simulink model "lunar_lander_sim_PWPF_transferMatrix_2023a"  (R2023a)
settings: Solver=FixedStepAuto  StartTime=0  StopTime=200  FixedStep=0.001  RelTol=1e-3
values from neighbouring files (symbols this model uses):
  D = Y_bar(:,1:m)    [Auxi_OKID_JXL.m]    (also in limit_cycle_est.m = 0:0.01:1)
undefined symbols (not defined in the file or in its folder): aMode
libraries: simulink_extras x8, slpidlib x6, shared6dofsys x2, sharedutil x2
settings Model: Creator=cnsl  LastModifiedBy=s3928

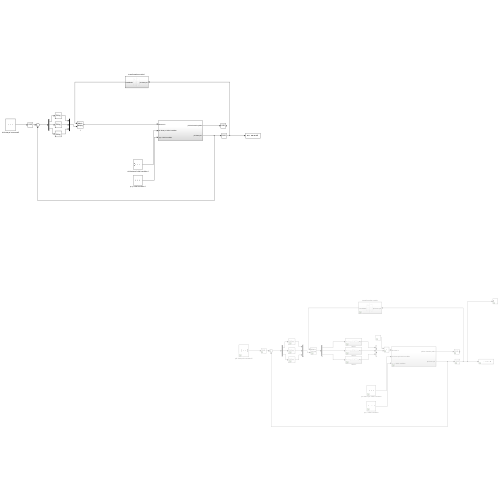
[thumbnail: Simulink's stored preview of the top-level diagram]
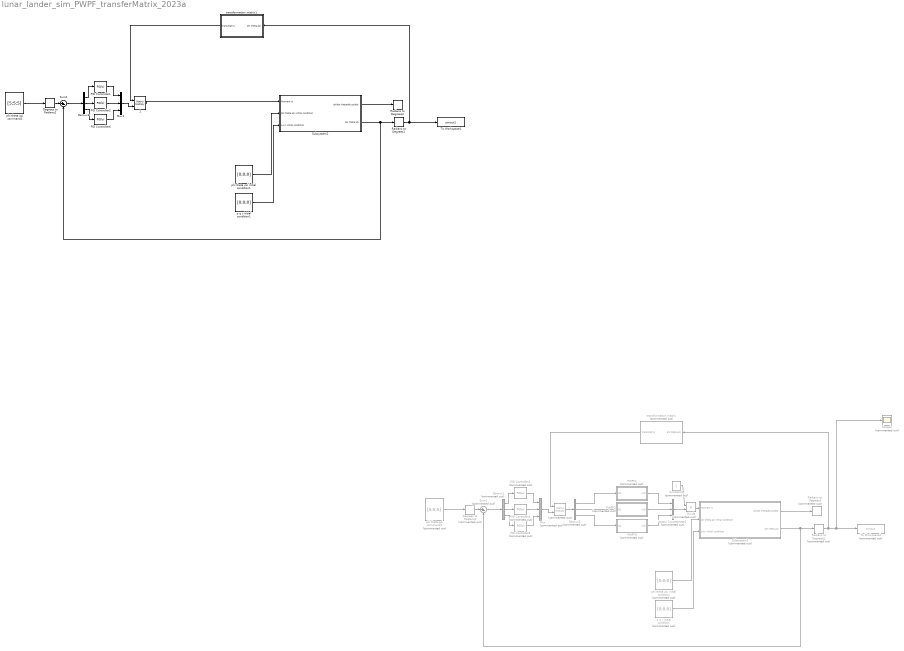
== system lunar_lander_sim_PWPF_transferMatrix_2023a ==
  " " : Product  Commented=on  Multiplication=Matrix(*)
  " 1" : Product  Multiplication=Matrix(*)
  " phi theta psi initial condition" : Constant  Commented=on  Value=[0;0;0]
  " phi theta psi initial condition1" : Constant  Value=[0;0;0]
  Constant1 : Constant  Commented=on
  Degrees to Radians1 : simulink_extras/Transformations/Degrees to Radians  Commented=on
  Degrees to Radians2 : simulink_extras/Transformations/Degrees to Radians
  Demux1 : Demux  Commented=on  Outputs=3
  Demux2 : Demux  Commented=on  Outputs=3
  Demux3 : Demux  Outputs=3
  Divide : Product  Commented=on  Inputs=**
  Mux : Mux  Commented=on  Inputs=3
  Mux1 : Mux  Inputs=3
  PID Controller1 : slpidlib/PID Controller  Controller=PID  Form=Parallel  TimeDomain=Continuous-time  UseExternalTs=off  SampleTime=-1  IntegratorMethod=Forward Euler  FilterMethod=Forward Euler  ControllerParametersSource=internal  P=6.69190722803613e+42  I=1.61303555234006e+36  UseKiTs=off  D=6.168461448375e+48  N=0.00472186710535811  UseFilter=on  TunerSelectOption=Transfer Function Based (PID Tuner App)  InitialConditionSource=internal  InitialConditionForIntegrator=0  InitialConditionForFilter=0  DifferentiatorICPrevScaledInput=0  ExternalReset=none  TrackingMode=off  Kt=1  LimitOutput=off  SatLimitsSource=internal  UpperSaturationLimit=inf  LowerSaturationLimit=-inf  LinearizeAsGain=on  AntiWindupMode=none  Kb=1  LimitIntegrator=off  UpperIntegratorSaturationLimit=inf  LowerIntegratorSaturationLimit=-inf  POutMin=[]  POutMax=[]  IOutMin=[]  IOutMax=[]  DOutMin=[]  DOutMax=[]  NOutMin=[]  NOutMax=[]  SumOutMin=[]  SumOutMax=[]  SaturationOutMin=[]  SaturationOutMax=[]  PParamMin=[]  PParamMax=[]  IParamMin=[]  IParamMax=[]  DParamMin=[]  DParamMax=[]  NParamMin=[]  NParamMax=[]  KbParamMin=[]  KbParamMax=[]  KtParamMin=[]  KtParamMax=[]  KbOutMin=[]  KbOutMax=[]  KtOutMin=[]  KtOutMax=[]  IntegratorOutMin=[]  IntegratorOutMax=[]  FilterOutMin=[]  FilterOutMax=[]  SumI1OutMin=[]  SumI1OutMax=[]  SumI2OutMin=[]  SumI2OutMax=[]  SumI3OutMin=[]  SumI3OutMax=[]  SumI4OutMin=[]  SumI4OutMax=[]  SumDOutMin=[]  SumDOutMax=[]  DifferentiatorOutMin=[]  DifferentiatorOutMax=[]  FilterDiffOutCoefMin=[]  FilterDiffOutCoefMax=[]  ReciprocalOutMin=[]  ReciprocalOutMax=[]  SumDenOutMin=[]  SumDenOutMax=[]  SumNumOutMin=[]  SumNumOutMax=[]  DivideOutMin=[]  DivideOutMax=[]  UdiffTsProdOutMin=[]  UdiffTsProdOutMax=[]  NTsProdOutMin=[]  NTsProdOutMax=[]  UintegralTsProdOutMin=[]  UintegralTsProdOutMax=[]  UngainTsProdOutMin=[]  UngainTsProdOutMax=[]  ClampingZeroOutDataTypeStr=Inherit: Inherit via back propagation  ClampingZeroOutMin=[]  ClampingZeroOutMax=[]  FilterDenConstantOutDataTypeStr=Inherit: Inherit via back propagation  FilterDenConstantOutMin=[]  FilterDenConstantOutMax=[]  PCopyOutDataTypeStr=Inherit: Inherit via back propagation  PCopyOutMin=[]  PCopyOutMax=[]  NCopyOutDataTypeStr=Inherit: Inherit via back propagation  NCopyOutMin=[]  NCopyOutMax=[]  IntegratorContinuousStateAttributes=''  IntegratorStateMustResolveToSignalObject=off  IntegratorRTWStateStorageClass=Auto  FilterContinuousStateAttributes=''  FilterStateMustResolveToSignalObject=off  FilterRTWStateStorageClass=Auto  ParallelPVariant=InternalParameters  IdealPVariant=Disabled  IVariant=InternalParameters  DVariant=InternalParameters  IntegratorVariant=Continuous  SatVariant=Disabled  AWVariant=Passthrough  PCopyVariant=Disabled  TRVariant=Disabled  FdbkBlocksVariant=Forward  IdealPFdbkVariant=Disabled  SatFdbkVariant=Disabled  DerivativeFilterVariant=ContFilter  NVariant=InternalParameters  NCopyVariant=Disabled  FilterICVariant=InternalICsFilter  IntegratorICVariant=InternalICs  ExternalResetVariant=Disabled  TRSumVariant=Passthrough  SumFdbkVariant=Disabled  SumVariant=Sum_PID  TsampFilterVariant=InternalTs  TsampNgainVariant=Passthrough  TsampIntegralVariant=Disabled_SignalSpec  ExternalSaturationOutDataTypeStr=Inherit: Same as second input
  PID Controller2 : slpidlib/PID Controller  Controller=PID  Form=Parallel  TimeDomain=Continuous-time  UseExternalTs=off  SampleTime=-1  IntegratorMethod=Forward Euler  FilterMethod=Forward Euler  ControllerParametersSource=internal  P=758060223807.445  I=15027742.3745305  UseKiTs=off  D=8.49639410270843e+15  N=0.388337887421907  UseFilter=on  TunerSelectOption=Transfer Function Based (PID Tuner App)  InitialConditionSource=internal  InitialConditionForIntegrator=0  InitialConditionForFilter=0  DifferentiatorICPrevScaledInput=0  ExternalReset=none  TrackingMode=off  Kt=1  LimitOutput=off  SatLimitsSource=internal  UpperSaturationLimit=inf  LowerSaturationLimit=-inf  LinearizeAsGain=on  AntiWindupMode=none  Kb=1  LimitIntegrator=off  UpperIntegratorSaturationLimit=inf  LowerIntegratorSaturationLimit=-inf  POutMin=[]  POutMax=[]  IOutMin=[]  IOutMax=[]  DOutMin=[]  DOutMax=[]  NOutMin=[]  NOutMax=[]  SumOutMin=[]  SumOutMax=[]  SaturationOutMin=[]  SaturationOutMax=[]  PParamMin=[]  PParamMax=[]  IParamMin=[]  IParamMax=[]  DParamMin=[]  DParamMax=[]  NParamMin=[]  NParamMax=[]  KbParamMin=[]  KbParamMax=[]  KtParamMin=[]  KtParamMax=[]  KbOutMin=[]  KbOutMax=[]  KtOutMin=[]  KtOutMax=[]  IntegratorOutMin=[]  IntegratorOutMax=[]  FilterOutMin=[]  FilterOutMax=[]  SumI1OutMin=[]  SumI1OutMax=[]  SumI2OutMin=[]  SumI2OutMax=[]  SumI3OutMin=[]  SumI3OutMax=[]  SumI4OutMin=[]  SumI4OutMax=[]  SumDOutMin=[]  SumDOutMax=[]  DifferentiatorOutMin=[]  DifferentiatorOutMax=[]  FilterDiffOutCoefMin=[]  FilterDiffOutCoefMax=[]  ReciprocalOutMin=[]  ReciprocalOutMax=[]  SumDenOutMin=[]  SumDenOutMax=[]  SumNumOutMin=[]  SumNumOutMax=[]  DivideOutMin=[]  DivideOutMax=[]  UdiffTsProdOutMin=[]  UdiffTsProdOutMax=[]  NTsProdOutMin=[]  NTsProdOutMax=[]  UintegralTsProdOutMin=[]  UintegralTsProdOutMax=[]  UngainTsProdOutMin=[]  UngainTsProdOutMax=[]  ClampingZeroOutDataTypeStr=Inherit: Inherit via back propagation  ClampingZeroOutMin=[]  ClampingZeroOutMax=[]  FilterDenConstantOutDataTypeStr=Inherit: Inherit via back propagation  FilterDenConstantOutMin=[]  FilterDenConstantOutMax=[]  PCopyOutDataTypeStr=Inherit: Inherit via back propagation  PCopyOutMin=[]  PCopyOutMax=[]  NCopyOutDataTypeStr=Inherit: Inherit via back propagation  NCopyOutMin=[]  NCopyOutMax=[]  IntegratorContinuousStateAttributes=''  IntegratorStateMustResolveToSignalObject=off  IntegratorRTWStateStorageClass=Auto  FilterContinuousStateAttributes=''  FilterStateMustResolveToSignalObject=off  FilterRTWStateStorageClass=Auto  ParallelPVariant=InternalParameters  IdealPVariant=Disabled  IVariant=InternalParameters  DVariant=InternalParameters  IntegratorVariant=Continuous  SatVariant=Disabled  AWVariant=Passthrough  PCopyVariant=Disabled  TRVariant=Disabled  FdbkBlocksVariant=Forward  IdealPFdbkVariant=Disabled  SatFdbkVariant=Disabled  DerivativeFilterVariant=ContFilter  NVariant=InternalParameters  NCopyVariant=Disabled  FilterICVariant=InternalICsFilter  IntegratorICVariant=InternalICs  ExternalResetVariant=Disabled  TRSumVariant=Passthrough  SumFdbkVariant=Disabled  SumVariant=Sum_PID  TsampFilterVariant=InternalTs  TsampNgainVariant=Passthrough  TsampIntegralVariant=Disabled_SignalSpec  ExternalSaturationOutDataTypeStr=Inherit: Same as second input
  PID Controller3 : slpidlib/PID Controller  Commented=on  Controller=PID  Form=Parallel  TimeDomain=Continuous-time  UseExternalTs=off  SampleTime=-1  IntegratorMethod=Forward Euler  FilterMethod=Forward Euler  ControllerParametersSource=internal  P=3  I=0.5  UseKiTs=off  D=8  N=1000  UseFilter=on  TunerSelectOption=Transfer Function Based (PID Tuner App)  InitialConditionSource=internal  InitialConditionForIntegrator=0  InitialConditionForFilter=0  DifferentiatorICPrevScaledInput=0  ExternalReset=none  TrackingMode=off  Kt=1  LimitOutput=off  SatLimitsSource=internal  UpperSaturationLimit=inf  LowerSaturationLimit=-inf  LinearizeAsGain=on  AntiWindupMode=none  Kb=1  LimitIntegrator=off  UpperIntegratorSaturationLimit=inf  LowerIntegratorSaturationLimit=-inf  POutMin=[]  POutMax=[]  IOutMin=[]  IOutMax=[]  DOutMin=[]  DOutMax=[]  NOutMin=[]  NOutMax=[]  SumOutMin=[]  SumOutMax=[]  SaturationOutMin=[]  SaturationOutMax=[]  PParamMin=[]  PParamMax=[]  IParamMin=[]  IParamMax=[]  DParamMin=[]  DParamMax=[]  NParamMin=[]  NParamMax=[]  KbParamMin=[]  KbParamMax=[]  KtParamMin=[]  KtParamMax=[]  KbOutMin=[]  KbOutMax=[]  KtOutMin=[]  KtOutMax=[]  IntegratorOutMin=[]  IntegratorOutMax=[]  FilterOutMin=[]  FilterOutMax=[]  SumI1OutMin=[]  SumI1OutMax=[]  SumI2OutMin=[]  SumI2OutMax=[]  SumI3OutMin=[]  SumI3OutMax=[]  SumI4OutMin=[]  SumI4OutMax=[]  SumDOutMin=[]  SumDOutMax=[]  DifferentiatorOutMin=[]  DifferentiatorOutMax=[]  FilterDiffOutCoefMin=[]  FilterDiffOutCoefMax=[]  ReciprocalOutMin=[]  ReciprocalOutMax=[]  SumDenOutMin=[]  SumDenOutMax=[]  SumNumOutMin=[]  SumNumOutMax=[]  DivideOutMin=[]  DivideOutMax=[]  UdiffTsProdOutMin=[]  UdiffTsProdOutMax=[]  NTsProdOutMin=[]  NTsProdOutMax=[]  UintegralTsProdOutMin=[]  UintegralTsProdOutMax=[]  UngainTsProdOutMin=[]  UngainTsProdOutMax=[]  ClampingZeroOutDataTypeStr=Inherit: Inherit via back propagation  ClampingZeroOutMin=[]  ClampingZeroOutMax=[]  FilterDenConstantOutDataTypeStr=Inherit: Inherit via back propagation  FilterDenConstantOutMin=[]  FilterDenConstantOutMax=[]  PCopyOutDataTypeStr=Inherit: Inherit via back propagation  PCopyOutMin=[]  PCopyOutMax=[]  NCopyOutDataTypeStr=Inherit: Inherit via back propagation  NCopyOutMin=[]  NCopyOutMax=[]  IntegratorContinuousStateAttributes=''  IntegratorStateMustResolveToSignalObject=off  IntegratorRTWStateStorageClass=Auto  FilterContinuousStateAttributes=''  FilterStateMustResolveToSignalObject=off  FilterRTWStateStorageClass=Auto  ParallelPVariant=InternalParameters  IdealPVariant=Disabled  IVariant=InternalParameters  DVariant=InternalParameters  IntegratorVariant=Continuous  SatVariant=Disabled  AWVariant=Passthrough  PCopyVariant=Disabled  TRVariant=Disabled  FdbkBlocksVariant=Forward  IdealPFdbkVariant=Disabled  SatFdbkVariant=Disabled  DerivativeFilterVariant=ContFilter  NVariant=InternalParameters  NCopyVariant=Disabled  FilterICVariant=InternalICsFilter  IntegratorICVariant=InternalICs  ExternalResetVariant=Disabled  TRSumVariant=Passthrough  SumFdbkVariant=Disabled  SumVariant=Sum_PID  TsampFilterVariant=InternalTs  TsampNgainVariant=Passthrough  TsampIntegralVariant=Disabled_SignalSpec  ExternalSaturationOutDataTypeStr=Inherit: Same as second input
  PID Controller4 : slpidlib/PID Controller  Commented=on  Controller=PID  Form=Parallel  TimeDomain=Continuous-time  UseExternalTs=off  SampleTime=-1  IntegratorMethod=Forward Euler  FilterMethod=Forward Euler  ControllerParametersSource=internal  P=2  I=0.1  UseKiTs=off  D=8  N=1000  UseFilter=on  TunerSelectOption=Transfer Function Based (PID Tuner App)  InitialConditionSource=internal  InitialConditionForIntegrator=0  InitialConditionForFilter=0  DifferentiatorICPrevScaledInput=0  ExternalReset=none  TrackingMode=off  Kt=1  LimitOutput=off  SatLimitsSource=internal  UpperSaturationLimit=inf  LowerSaturationLimit=-inf  LinearizeAsGain=on  AntiWindupMode=none  Kb=1  LimitIntegrator=off  UpperIntegratorSaturationLimit=inf  LowerIntegratorSaturationLimit=-inf  POutMin=[]  POutMax=[]  IOutMin=[]  IOutMax=[]  DOutMin=[]  DOutMax=[]  NOutMin=[]  NOutMax=[]  SumOutMin=[]  SumOutMax=[]  SaturationOutMin=[]  SaturationOutMax=[]  PParamMin=[]  PParamMax=[]  IParamMin=[]  IParamMax=[]  DParamMin=[]  DParamMax=[]  NParamMin=[]  NParamMax=[]  KbParamMin=[]  KbParamMax=[]  KtParamMin=[]  KtParamMax=[]  KbOutMin=[]  KbOutMax=[]  KtOutMin=[]  KtOutMax=[]  IntegratorOutMin=[]  IntegratorOutMax=[]  FilterOutMin=[]  FilterOutMax=[]  SumI1OutMin=[]  SumI1OutMax=[]  SumI2OutMin=[]  SumI2OutMax=[]  SumI3OutMin=[]  SumI3OutMax=[]  SumI4OutMin=[]  SumI4OutMax=[]  SumDOutMin=[]  SumDOutMax=[]  DifferentiatorOutMin=[]  DifferentiatorOutMax=[]  FilterDiffOutCoefMin=[]  FilterDiffOutCoefMax=[]  ReciprocalOutMin=[]  ReciprocalOutMax=[]  SumDenOutMin=[]  SumDenOutMax=[]  SumNumOutMin=[]  SumNumOutMax=[]  DivideOutMin=[]  DivideOutMax=[]  UdiffTsProdOutMin=[]  UdiffTsProdOutMax=[]  NTsProdOutMin=[]  NTsProdOutMax=[]  UintegralTsProdOutMin=[]  UintegralTsProdOutMax=[]  UngainTsProdOutMin=[]  UngainTsProdOutMax=[]  ClampingZeroOutDataTypeStr=Inherit: Inherit via back propagation  ClampingZeroOutMin=[]  ClampingZeroOutMax=[]  FilterDenConstantOutDataTypeStr=Inherit: Inherit via back propagation  FilterDenConstantOutMin=[]  FilterDenConstantOutMax=[]  PCopyOutDataTypeStr=Inherit: Inherit via back propagation  PCopyOutMin=[]  PCopyOutMax=[]  NCopyOutDataTypeStr=Inherit: Inherit via back propagation  NCopyOutMin=[]  NCopyOutMax=[]  IntegratorContinuousStateAttributes=''  IntegratorStateMustResolveToSignalObject=off  IntegratorRTWStateStorageClass=Auto  FilterContinuousStateAttributes=''  FilterStateMustResolveToSignalObject=off  FilterRTWStateStorageClass=Auto  ParallelPVariant=InternalParameters  IdealPVariant=Disabled  IVariant=InternalParameters  DVariant=InternalParameters  IntegratorVariant=Continuous  SatVariant=Disabled  AWVariant=Passthrough  PCopyVariant=Disabled  TRVariant=Disabled  FdbkBlocksVariant=Forward  IdealPFdbkVariant=Disabled  SatFdbkVariant=Disabled  DerivativeFilterVariant=ContFilter  NVariant=InternalParameters  NCopyVariant=Disabled  FilterICVariant=InternalICsFilter  IntegratorICVariant=InternalICs  ExternalResetVariant=Disabled  TRSumVariant=Passthrough  SumFdbkVariant=Disabled  SumVariant=Sum_PID  TsampFilterVariant=InternalTs  TsampNgainVariant=Passthrough  TsampIntegralVariant=Disabled_SignalSpec  ExternalSaturationOutDataTypeStr=Inherit: Same as second input
  PID Controller5 : slpidlib/PID Controller  Commented=on  Controller=PID  Form=Parallel  TimeDomain=Continuous-time  UseExternalTs=off  SampleTime=-1  IntegratorMethod=Forward Euler  FilterMethod=Forward Euler  ControllerParametersSource=internal  P=3  I=0.2  UseKiTs=off  D=12  N=1000  UseFilter=on  TunerSelectOption=Transfer Function Based (PID Tuner App)  InitialConditionSource=internal  InitialConditionForIntegrator=0  InitialConditionForFilter=0  DifferentiatorICPrevScaledInput=0  ExternalReset=none  TrackingMode=off  Kt=1  LimitOutput=off  SatLimitsSource=internal  UpperSaturationLimit=inf  LowerSaturationLimit=-inf  LinearizeAsGain=on  AntiWindupMode=none  Kb=1  LimitIntegrator=off  UpperIntegratorSaturationLimit=inf  LowerIntegratorSaturationLimit=-inf  POutMin=[]  POutMax=[]  IOutMin=[]  IOutMax=[]  DOutMin=[]  DOutMax=[]  NOutMin=[]  NOutMax=[]  SumOutMin=[]  SumOutMax=[]  SaturationOutMin=[]  SaturationOutMax=[]  PParamMin=[]  PParamMax=[]  IParamMin=[]  IParamMax=[]  DParamMin=[]  DParamMax=[]  NParamMin=[]  NParamMax=[]  KbParamMin=[]  KbParamMax=[]  KtParamMin=[]  KtParamMax=[]  KbOutMin=[]  KbOutMax=[]  KtOutMin=[]  KtOutMax=[]  IntegratorOutMin=[]  IntegratorOutMax=[]  FilterOutMin=[]  FilterOutMax=[]  SumI1OutMin=[]  SumI1OutMax=[]  SumI2OutMin=[]  SumI2OutMax=[]  SumI3OutMin=[]  SumI3OutMax=[]  SumI4OutMin=[]  SumI4OutMax=[]  SumDOutMin=[]  SumDOutMax=[]  DifferentiatorOutMin=[]  DifferentiatorOutMax=[]  FilterDiffOutCoefMin=[]  FilterDiffOutCoefMax=[]  ReciprocalOutMin=[]  ReciprocalOutMax=[]  SumDenOutMin=[]  SumDenOutMax=[]  SumNumOutMin=[]  SumNumOutMax=[]  DivideOutMin=[]  DivideOutMax=[]  UdiffTsProdOutMin=[]  UdiffTsProdOutMax=[]  NTsProdOutMin=[]  NTsProdOutMax=[]  UintegralTsProdOutMin=[]  UintegralTsProdOutMax=[]  UngainTsProdOutMin=[]  UngainTsProdOutMax=[]  ClampingZeroOutDataTypeStr=Inherit: Inherit via back propagation  ClampingZeroOutMin=[]  ClampingZeroOutMax=[]  FilterDenConstantOutDataTypeStr=Inherit: Inherit via back propagation  FilterDenConstantOutMin=[]  FilterDenConstantOutMax=[]  PCopyOutDataTypeStr=Inherit: Inherit via back propagation  PCopyOutMin=[]  PCopyOutMax=[]  NCopyOutDataTypeStr=Inherit: Inherit via back propagation  NCopyOutMin=[]  NCopyOutMax=[]  IntegratorContinuousStateAttributes=''  IntegratorStateMustResolveToSignalObject=off  IntegratorRTWStateStorageClass=Auto  FilterContinuousStateAttributes=''  FilterStateMustResolveToSignalObject=off  FilterRTWStateStorageClass=Auto  ParallelPVariant=InternalParameters  IdealPVariant=Disabled  IVariant=InternalParameters  DVariant=InternalParameters  IntegratorVariant=Continuous  SatVariant=Disabled  AWVariant=Passthrough  PCopyVariant=Disabled  TRVariant=Disabled  FdbkBlocksVariant=Forward  IdealPFdbkVariant=Disabled  SatFdbkVariant=Disabled  DerivativeFilterVariant=ContFilter  NVariant=InternalParameters  NCopyVariant=Disabled  FilterICVariant=InternalICsFilter  IntegratorICVariant=InternalICs  ExternalResetVariant=Disabled  TRSumVariant=Passthrough  SumFdbkVariant=Disabled  SumVariant=Sum_PID  TsampFilterVariant=InternalTs  TsampNgainVariant=Passthrough  TsampIntegralVariant=Disabled_SignalSpec  ExternalSaturationOutDataTypeStr=Inherit: Same as second input
  PID Controller6 : slpidlib/PID Controller  Controller=PID  Form=Parallel  TimeDomain=Continuous-time  UseExternalTs=off  SampleTime=-1  IntegratorMethod=Forward Euler  FilterMethod=Forward Euler  ControllerParametersSource=internal  P=6.22138293474319e+23  I=1.51651183268484e+18  UseKiTs=off  D=5.67086142970331e+28  N=0.0477505745520356  UseFilter=on  TunerSelectOption=Transfer Function Based (PID Tuner App)  InitialConditionSource=internal  InitialConditionForIntegrator=0  InitialConditionForFilter=0  DifferentiatorICPrevScaledInput=0  ExternalReset=none  TrackingMode=off  Kt=1  LimitOutput=off  SatLimitsSource=internal  UpperSaturationLimit=inf  LowerSaturationLimit=-inf  LinearizeAsGain=on  AntiWindupMode=none  Kb=1  LimitIntegrator=off  UpperIntegratorSaturationLimit=inf  LowerIntegratorSaturationLimit=-inf  POutMin=[]  POutMax=[]  IOutMin=[]  IOutMax=[]  DOutMin=[]  DOutMax=[]  NOutMin=[]  NOutMax=[]  SumOutMin=[]  SumOutMax=[]  SaturationOutMin=[]  SaturationOutMax=[]  PParamMin=[]  PParamMax=[]  IParamMin=[]  IParamMax=[]  DParamMin=[]  DParamMax=[]  NParamMin=[]  NParamMax=[]  KbParamMin=[]  KbParamMax=[]  KtParamMin=[]  KtParamMax=[]  KbOutMin=[]  KbOutMax=[]  KtOutMin=[]  KtOutMax=[]  IntegratorOutMin=[]  IntegratorOutMax=[]  FilterOutMin=[]  FilterOutMax=[]  SumI1OutMin=[]  SumI1OutMax=[]  SumI2OutMin=[]  SumI2OutMax=[]  SumI3OutMin=[]  SumI3OutMax=[]  SumI4OutMin=[]  SumI4OutMax=[]  SumDOutMin=[]  SumDOutMax=[]  DifferentiatorOutMin=[]  DifferentiatorOutMax=[]  FilterDiffOutCoefMin=[]  FilterDiffOutCoefMax=[]  ReciprocalOutMin=[]  ReciprocalOutMax=[]  SumDenOutMin=[]  SumDenOutMax=[]  SumNumOutMin=[]  SumNumOutMax=[]  DivideOutMin=[]  DivideOutMax=[]  UdiffTsProdOutMin=[]  UdiffTsProdOutMax=[]  NTsProdOutMin=[]  NTsProdOutMax=[]  UintegralTsProdOutMin=[]  UintegralTsProdOutMax=[]  UngainTsProdOutMin=[]  UngainTsProdOutMax=[]  ClampingZeroOutDataTypeStr=Inherit: Inherit via back propagation  ClampingZeroOutMin=[]  ClampingZeroOutMax=[]  FilterDenConstantOutDataTypeStr=Inherit: Inherit via back propagation  FilterDenConstantOutMin=[]  FilterDenConstantOutMax=[]  PCopyOutDataTypeStr=Inherit: Inherit via back propagation  PCopyOutMin=[]  PCopyOutMax=[]  NCopyOutDataTypeStr=Inherit: Inherit via back propagation  NCopyOutMin=[]  NCopyOutMax=[]  IntegratorContinuousStateAttributes=''  IntegratorStateMustResolveToSignalObject=off  IntegratorRTWStateStorageClass=Auto  FilterContinuousStateAttributes=''  FilterStateMustResolveToSignalObject=off  FilterRTWStateStorageClass=Auto  ParallelPVariant=InternalParameters  IdealPVariant=Disabled  IVariant=InternalParameters  DVariant=InternalParameters  IntegratorVariant=Continuous  SatVariant=Disabled  AWVariant=Passthrough  PCopyVariant=Disabled  TRVariant=Disabled  FdbkBlocksVariant=Forward  IdealPFdbkVariant=Disabled  SatFdbkVariant=Disabled  DerivativeFilterVariant=ContFilter  NVariant=InternalParameters  NCopyVariant=Disabled  FilterICVariant=InternalICsFilter  IntegratorICVariant=InternalICs  ExternalResetVariant=Disabled  TRSumVariant=Passthrough  SumFdbkVariant=Disabled  SumVariant=Sum_PID  TsampFilterVariant=InternalTs  TsampNgainVariant=Passthrough  TsampIntegralVariant=Disabled_SignalSpec  ExternalSaturationOutDataTypeStr=Inherit: Same as second input
  PWPF1 : Subsystem  Commented=on
  PWPF2 : Subsystem  Commented=on
  PWPF3 : Subsystem  Commented=on
  Radians to Degrees1 : simulink_extras/Transformations/Radians to Degrees
  Radians to Degrees2 : simulink_extras/Transformations/Radians to Degrees  Commented=on
  Radians to Degrees3 : simulink_extras/Transformations/Radians to Degrees  Commented=on
  Radians to Degrees4 : simulink_extras/Transformations/Radians to Degrees
  Scope3 : Scope  Commented=on
  Subsystem1 : Subsystem  Commented=on
  Subsystem2 : Subsystem
  Sum1 : Sum  Commented=on  Inputs=|+-
  Sum2 : Sum  Inputs=|+-
  To Workspace1 : ToWorkspace  VariableName=simout1  SaveFormat=Timeseries  SampleTime=-1
  To Workspace3 : ToWorkspace  Commented=on  VariableName=simout  SaveFormat=Timeseries  SampleTime=-1
  Vector Concatenate1 : Concatenate  Commented=on  NumInputs=3
  p q r initial condition : Constant  Commented=on  Value=[0;0;0]
  p q r initial condition1 : Constant  Value=[0;0;0]
  phi theta psi command1 : Constant  Commented=on  Value=[5;5;5]
  phi theta psi command2 : Constant  Value=[5;5;5]
  transformation matrix : Subsystem  Commented=on
  transformation matrix1 : Subsystem
  wires:
  Sum1/1 -> Demux1/1
  phi theta psi command1/1 -> Degrees to Radians1/1
  Demux1/2 -> PID Controller4/1
  Demux1/3 -> PID Controller5/1
  Subsystem1/1(phidot thetadot psidot) -> Radians to Degrees3/1
  Demux1/1 -> PID Controller3/1
  Degrees to Radians1/1 -> Sum1/1
  Radians to Degrees2/1 -> Scope3/1, To Workspace3/1, transformation matrix/1(phi theta psi)
  " phi theta psi initial condition"/1 -> Subsystem1/2("phi theta psi initial condition ")
  Subsystem1/2("phi theta psi ") -> Sum1/2, Radians to Degrees2/1
  p q r initial condition/1 -> Subsystem1/3(" p q r initial condition")
  PWPF2/1(u(t)) -> Vector Concatenate1/2
  PWPF3/1(u(t)) -> Vector Concatenate1/3
  PWPF1/1(u(t)) -> Vector Concatenate1/1
  Vector Concatenate1/1 -> Divide/2
  Constant1/1 -> Divide/1
  transformation matrix/1(transMatrix) -> " "/1
  Divide/1 -> Subsystem1/1(Moment in)
  PID Controller4/1 -> Mux/2
  PID Controller3/1 -> Mux/1
  PID Controller5/1 -> Mux/3
  Mux/1 -> " "/2
  " "/1 -> Demux2/1
  Demux2/1 -> PWPF1/1(In1)
  Demux2/2 -> PWPF2/1(In1)
  Demux2/3 -> PWPF3/1(In1)
  PID Controller1/1 -> Mux1/1
  Mux1/1 -> " 1"/2
  transformation matrix1/1(transMatrix) -> " 1"/1
  Demux3/3 -> PID Controller6/1
  Radians to Degrees1/1 -> To Workspace1/1, transformation matrix1/1(phi theta psi)
  p q r initial condition1/1 -> Subsystem2/3(" p q r initial condition")
  Demux3/1 -> PID Controller1/1
  PID Controller2/1 -> Mux1/2
  Degrees to Radians2/1 -> Sum2/1
  " phi theta psi initial condition1"/1 -> Subsystem2/2("phi theta psi initial condition ")
  phi theta psi command2/1 -> Degrees to Radians2/1
  Sum2/1 -> Demux3/1
  Demux3/2 -> PID Controller2/1
  Subsystem2/2("phi theta psi ") -> Sum2/2, Radians to Degrees1/1
  PID Controller6/1 -> Mux1/3
  Subsystem2/1(phidot thetadot psidot) -> Radians to Degrees4/1
  " 1"/1 -> Subsystem2/1(Moment in)

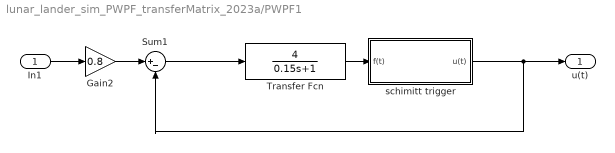
== system lunar_lander_sim_PWPF_transferMatrix_2023a/PWPF1 ==
  In1 : Inport
  Gain2 : Gain  Gain=0.8
  Sum1 : Sum  Inputs=|+-
  Transfer Fcn : TransferFcn  Numerator=[4]  Denominator=[0.15 1]
  schimitt trigger : Subsystem
  u(t) : Outport
  wires:
  Transfer Fcn/1 -> schimitt trigger/1(f(t))
  Sum1/1 -> Transfer Fcn/1
  schimitt trigger/1(u(t)) -> Sum1/2, u(t)/1
  Gain2/1 -> Sum1/1
  In1/1 -> Gain2/1

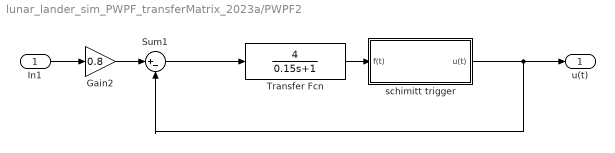
== system lunar_lander_sim_PWPF_transferMatrix_2023a/PWPF2 ==
  In1 : Inport
  Gain2 : Gain  Gain=0.8
  Sum1 : Sum  Inputs=|+-
  Transfer Fcn : TransferFcn  Numerator=[4]  Denominator=[0.15 1]
  schimitt trigger : Subsystem
  u(t) : Outport
  wires:
  In1/1 -> Gain2/1
  Gain2/1 -> Sum1/1
  schimitt trigger/1(u(t)) -> u(t)/1, Sum1/2
  Sum1/1 -> Transfer Fcn/1
  Transfer Fcn/1 -> schimitt trigger/1(f(t))

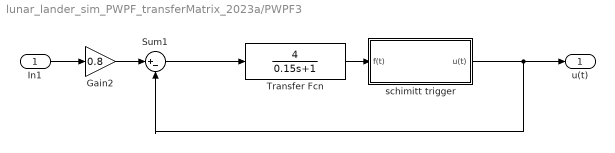
== system lunar_lander_sim_PWPF_transferMatrix_2023a/PWPF3 ==
  In1 : Inport
  Gain2 : Gain  Gain=0.8
  Sum1 : Sum  Inputs=|+-
  Transfer Fcn : TransferFcn  Numerator=[4]  Denominator=[0.15 1]
  schimitt trigger : Subsystem
  u(t) : Outport
  wires:
  Transfer Fcn/1 -> schimitt trigger/1(f(t))
  Sum1/1 -> Transfer Fcn/1
  schimitt trigger/1(u(t)) -> Sum1/2, u(t)/1
  Gain2/1 -> Sum1/1
  In1/1 -> Gain2/1

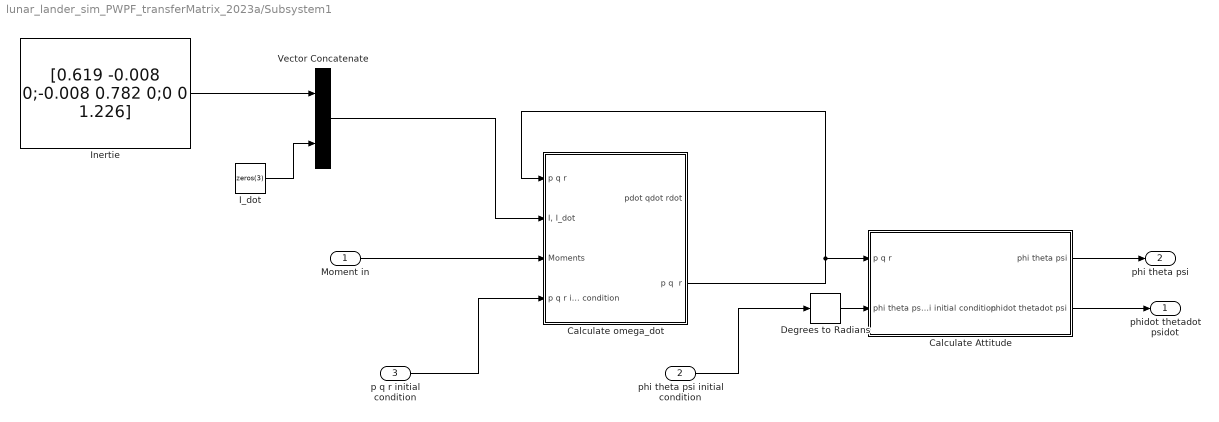
== system lunar_lander_sim_PWPF_transferMatrix_2023a/Subsystem1 ==
  Moment in : Inport
  "phi theta psi initial condition " : Inport  Port=2
  " p q r initial condition" : Inport  Port=3
  "Calculate Attitude " : Subsystem
  Calculate omega_dot : Subsystem  AncestorBlock=shared6dofsys/Calculate omega_dot  mask{aMode=aMode}
      mask init:
      | if aerosharedtest(gcb)
      |     aerosharedicon('shared');
      | else
      |     sharedautoicon('shared');
      | end
      settings: LibrarySourceBlock=shared6dofsys/Calculate omega_dot
  Degrees to Radians : simulink_extras/Transformations/Degrees to Radians
  I_dot : Constant  Value=zeros(3)
  Inertie : Constant  Value=[0.619 -0.008 0;-0.008 0.782 0;0 0 1.226]
  Vector Concatenate : Concatenate  Mode=Multidimensional array
  phidot thetadot psidot : Outport
  "phi theta psi " : Outport  Port=2
  wires:
  Vector Concatenate/1 -> Calculate omega_dot/2("I, I_dot")
  Inertie/1 -> Vector Concatenate/1
  Calculate omega_dot/2(p q  r) -> Calculate omega_dot/1(p q r), "Calculate Attitude "/1(p q r)
  I_dot/1 -> Vector Concatenate/2
  " p q r initial condition"/1 -> Calculate omega_dot/4(p q r initial condition)
  "Calculate Attitude "/1("phi theta psi ") -> "phi theta psi "/1
  Degrees to Radians/1 -> "Calculate Attitude "/2("phi theta psi initial condition ")
  "phi theta psi initial condition "/1 -> Degrees to Radians/1
  "Calculate Attitude "/2(phidot thetadot psi) -> phidot thetadot psidot/1
  Moment in/1 -> Calculate omega_dot/3(Moments)

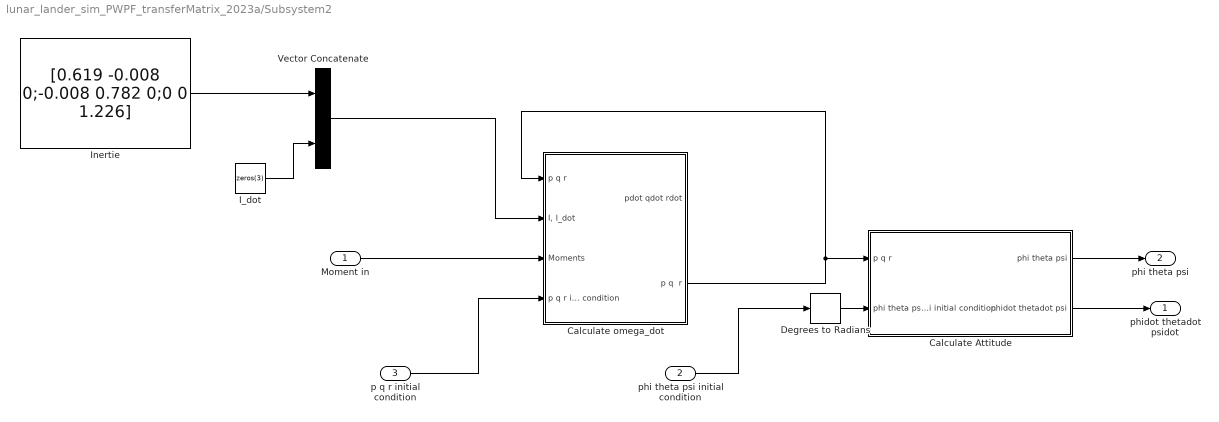
== system lunar_lander_sim_PWPF_transferMatrix_2023a/Subsystem2 ==
  Moment in : Inport
  "phi theta psi initial condition " : Inport  Port=2
  " p q r initial condition" : Inport  Port=3
  "Calculate Attitude " : Subsystem
  Calculate omega_dot : Subsystem  AncestorBlock=shared6dofsys/Calculate omega_dot  mask{aMode=aMode}
      mask init:
      | if aerosharedtest(gcb)
      |     aerosharedicon('shared');
      | else
      |     sharedautoicon('shared');
      | end
      settings: LibrarySourceBlock=shared6dofsys/Calculate omega_dot
  Degrees to Radians : simulink_extras/Transformations/Degrees to Radians
  I_dot : Constant  Value=zeros(3)
  Inertie : Constant  Value=[0.619 -0.008 0;-0.008 0.782 0;0 0 1.226]
  Vector Concatenate : Concatenate  Mode=Multidimensional array
  phidot thetadot psidot : Outport
  "phi theta psi " : Outport  Port=2
  wires:
  Vector Concatenate/1 -> Calculate omega_dot/2("I, I_dot")
  Inertie/1 -> Vector Concatenate/1
  Calculate omega_dot/2(p q  r) -> Calculate omega_dot/1(p q r), "Calculate Attitude "/1(p q r)
  I_dot/1 -> Vector Concatenate/2
  " p q r initial condition"/1 -> Calculate omega_dot/4(p q r initial condition)
  "Calculate Attitude "/1("phi theta psi ") -> "phi theta psi "/1
  Degrees to Radians/1 -> "Calculate Attitude "/2("phi theta psi initial condition ")
  "phi theta psi initial condition "/1 -> Degrees to Radians/1
  "Calculate Attitude "/2(phidot thetadot psi) -> phidot thetadot psidot/1
  Moment in/1 -> Calculate omega_dot/3(Moments)

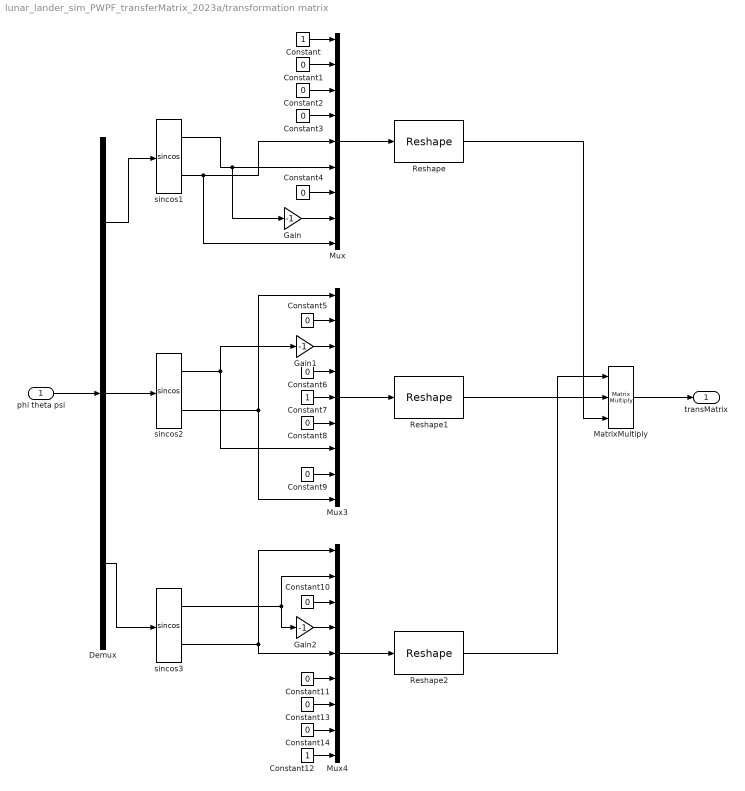
== system lunar_lander_sim_PWPF_transferMatrix_2023a/transformation matrix ==
  phi theta psi : Inport
  Constant : Constant
  Constant{1..6,8..11,13..14} (12 alike) : Constant  Value=0
  Constant12 : Constant
  Constant7 : Constant
  Demux : Demux  Outputs=3
  Gain : Gain  Gain=-1
  Gain1 : Gain  Gain=-1
  Gain2 : Gain  Gain=-1
  MatrixMultiply : Product  Inputs=3  Multiplication=Matrix(*)
  Mux : Mux  Inputs=9
  Mux3 : Mux  Inputs=9
  Mux4 : Mux  Inputs=9
  Reshape : Reshape  OutputDimensionality=Customize  OutputDimensions=[3,3]
  Reshape1 : Reshape  OutputDimensionality=Customize  OutputDimensions=[3,3]
  Reshape2 : Reshape  OutputDimensionality=Customize  OutputDimensions=[3,3]
  sincos1 : Trigonometry  Operator=sincos
  sincos2 : Trigonometry  Operator=sincos
  sincos3 : Trigonometry  Operator=sincos
  transMatrix : Outport
  wires:
  phi theta psi/1 -> Demux/1
  Demux/1 -> sincos1/1
  Demux/2 -> sincos2/1
  Demux/3 -> sincos3/1
  Mux/1 -> Reshape/1
  Constant/1 -> Mux/1
  Constant1/1 -> Mux/2
  Constant2/1 -> Mux/3
  Constant3/1 -> Mux/4
  sincos1/2 -> Mux/9, Mux/5
  sincos1/1 -> Gain/1, Mux/6
  Constant4/1 -> Mux/7
  Gain/1 -> Mux/8
  Mux3/1 -> Reshape1/1
  sincos2/2 -> Mux3/1, Mux3/9
  Constant5/1 -> Mux3/2
  sincos2/1 -> Gain1/1, Mux3/7
  Gain1/1 -> Mux3/3
  Constant6/1 -> Mux3/4
  Constant7/1 -> Mux3/5
  Constant8/1 -> Mux3/6
  Constant9/1 -> Mux3/8
  Mux4/1 -> Reshape2/1
  sincos3/2 -> Mux4/1, Mux4/5
  sincos3/1 -> Gain2/1, Mux4/2
  Constant10/1 -> Mux4/3
  Gain2/1 -> Mux4/4
  Constant11/1 -> Mux4/6
  Constant12/1 -> Mux4/9
  Constant13/1 -> Mux4/7
  Constant14/1 -> Mux4/8
  Reshape2/1 -> MatrixMultiply/1
  Reshape1/1 -> MatrixMultiply/2
  Reshape/1 -> MatrixMultiply/3
  MatrixMultiply/1 -> transMatrix/1

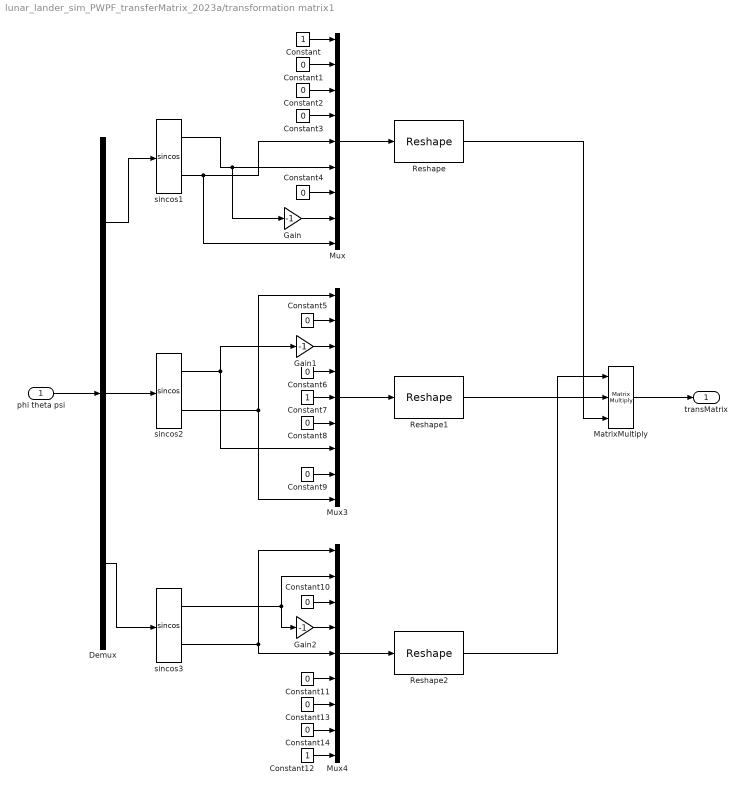
== system lunar_lander_sim_PWPF_transferMatrix_2023a/transformation matrix1 ==
  phi theta psi : Inport
  Constant : Constant
  Constant{1..6,8..11,13..14} (12 alike) : Constant  Value=0
  Constant12 : Constant
  Constant7 : Constant
  Demux : Demux  Outputs=3
  Gain : Gain  Gain=-1
  Gain1 : Gain  Gain=-1
  Gain2 : Gain  Gain=-1
  MatrixMultiply : Product  Inputs=3  Multiplication=Matrix(*)
  Mux : Mux  Inputs=9
  Mux3 : Mux  Inputs=9
  Mux4 : Mux  Inputs=9
  Reshape : Reshape  OutputDimensionality=Customize  OutputDimensions=[3,3]
  Reshape1 : Reshape  OutputDimensionality=Customize  OutputDimensions=[3,3]
  Reshape2 : Reshape  OutputDimensionality=Customize  OutputDimensions=[3,3]
  sincos1 : Trigonometry  Operator=sincos
  sincos2 : Trigonometry  Operator=sincos
  sincos3 : Trigonometry  Operator=sincos
  transMatrix : Outport
  wires:
  phi theta psi/1 -> Demux/1
  Demux/1 -> sincos1/1
  Demux/2 -> sincos2/1
  Demux/3 -> sincos3/1
  Mux/1 -> Reshape/1
  Constant/1 -> Mux/1
  Constant1/1 -> Mux/2
  Constant2/1 -> Mux/3
  Constant3/1 -> Mux/4
  sincos1/2 -> Mux/9, Mux/5
  sincos1/1 -> Gain/1, Mux/6
  Constant4/1 -> Mux/7
  Gain/1 -> Mux/8
  Mux3/1 -> Reshape1/1
  sincos2/2 -> Mux3/1, Mux3/9
  Constant5/1 -> Mux3/2
  sincos2/1 -> Gain1/1, Mux3/7
  Gain1/1 -> Mux3/3
  Constant6/1 -> Mux3/4
  Constant7/1 -> Mux3/5
  Constant8/1 -> Mux3/6
  Constant9/1 -> Mux3/8
  Mux4/1 -> Reshape2/1
  sincos3/2 -> Mux4/1, Mux4/5
  sincos3/1 -> Gain2/1, Mux4/2
  Constant10/1 -> Mux4/3
  Gain2/1 -> Mux4/4
  Constant11/1 -> Mux4/6
  Constant12/1 -> Mux4/9
  Constant13/1 -> Mux4/7
  Constant14/1 -> Mux4/8
  Reshape2/1 -> MatrixMultiply/1
  Reshape1/1 -> MatrixMultiply/2
  Reshape/1 -> MatrixMultiply/3
  MatrixMultiply/1 -> transMatrix/1

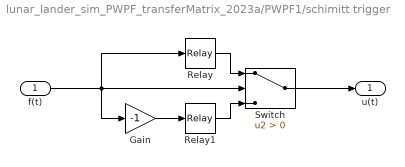
== system lunar_lander_sim_PWPF_transferMatrix_2023a/PWPF1/schimitt trigger ==
  f(t) : Inport
  Gain : Gain  Gain=-1
  Relay : Relay  OnSwitchValue=0.5  OffSwitchValue=0.15  OnOutputValue=4.5
  Relay1 : Relay  OnSwitchValue=0.5  OffSwitchValue=0.15  OnOutputValue=-4.5
  Switch : Switch  Criteria=u2 > Threshold  SaturateOnIntegerOverflow=off  InputSameDT=off
  u(t) : Outport
  wires:
  f(t)/1 -> Relay/1, Gain/1, Switch/2
  Relay1/1 -> Switch/3
  Gain/1 -> Relay1/1
  Relay/1 -> Switch/1
  Switch/1 -> u(t)/1

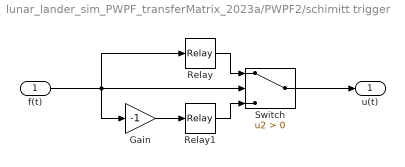
== system lunar_lander_sim_PWPF_transferMatrix_2023a/PWPF2/schimitt trigger ==
  f(t) : Inport
  Gain : Gain  Gain=-1
  Relay : Relay  OnSwitchValue=0.5  OffSwitchValue=0.15  OnOutputValue=4.5
  Relay1 : Relay  OnSwitchValue=0.5  OffSwitchValue=0.15  OnOutputValue=-4.5
  Switch : Switch  Criteria=u2 > Threshold  SaturateOnIntegerOverflow=off  InputSameDT=off
  u(t) : Outport
  wires:
  Switch/1 -> u(t)/1
  Relay/1 -> Switch/1
  Gain/1 -> Relay1/1
  Relay1/1 -> Switch/3
  f(t)/1 -> Switch/2, Gain/1, Relay/1

== system lunar_lander_sim_PWPF_transferMatrix_2023a/PWPF3/schimitt trigger ==
  f(t) : Inport
  Gain : Gain  Gain=-1
  Relay : Relay  OnSwitchValue=0.5  OffSwitchValue=0.15  OnOutputValue=4.5
  Relay1 : Relay  OnSwitchValue=0.5  OffSwitchValue=0.15  OnOutputValue=-4.5
  Switch : Switch  Criteria=u2 > Threshold  SaturateOnIntegerOverflow=off  InputSameDT=off
  u(t) : Outport
  wires:
  f(t)/1 -> Relay/1, Gain/1, Switch/2
  Relay1/1 -> Switch/3
  Gain/1 -> Relay1/1
  Relay/1 -> Switch/1
  Switch/1 -> u(t)/1

== system lunar_lander_sim_PWPF_transferMatrix_2023a/Subsystem1/Calculate Attitude  ==
  p q r : Inport
  "phi theta psi initial condition " : Inport  Port=2
  " " : Integrator  InitialConditionSource=external
  phidot thetadot psidot : shared6dofsys/DCM & Euler Angles (Euler)/phidot thetadot psidot  SystemSampleTime=-1  VariantActivationTime=update diagram  Latency=0  AutoFrameSizeCalculation=off
  "phi theta psi " : Outport
  phidot thetadot psi : Outport  Port=2
  wires:
  "phi theta psi initial condition "/1 -> " "/2
  " "/1 -> phidot thetadot psidot/2, "phi theta psi "/1
  phidot thetadot psidot/1 -> phidot thetadot psi/1, " "/1
  p q r/1 -> phidot thetadot psidot/1

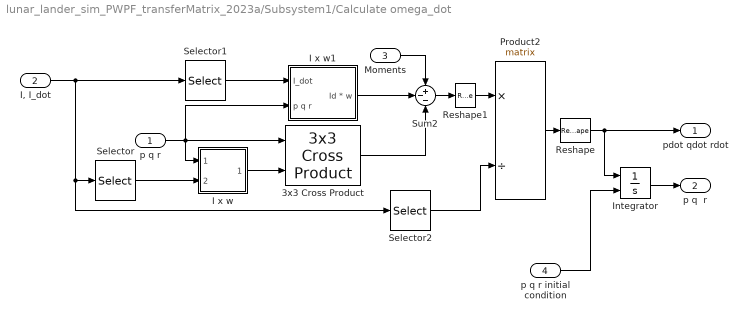
== system lunar_lander_sim_PWPF_transferMatrix_2023a/Subsystem1/Calculate omega_dot ==
  p q r : Inport  OutDataTypeStr=double
  "I, I_dot" : Inport  Port=2  OutDataTypeStr=double
  Moments : Inport  Port=3  OutDataTypeStr=double
  p q r initial condition : Inport  Port=4
  3x3 Cross Product : sharedutil/3x3 Cross Product  aMode=aMode
  I x w : Subsystem
  I x w1 : Subsystem
  Integrator : Integrator  InitialConditionSource=external
  Product2 : Product  Inputs=*/  Multiplication=Matrix(*)  SaturateOnIntegerOverflow=on  OutDataTypeStr=Inherit: Same as first input
  Reshape : Reshape
  Reshape1 : Reshape  OutputDimensionality=Row vector (2-D)
  Selector : Selector  NumberOfDimensions=2  InputPortWidth=2  IndexOptions=Index vector (dialog),Select all  Indices=1:3,-1  OutputSizes=1
  Selector1 : Selector  NumberOfDimensions=2  InputPortWidth=2  IndexOptions=Index vector (dialog),Select all  Indices=4:6,-1  OutputSizes=1
  Selector2 : Selector  NumberOfDimensions=2  InputPortWidth=2  IndexOptions=Index vector (dialog),Select all  Indices=1:3,-1  OutputSizes=1
  Sum2 : Sum  Inputs=+--  SaturateOnIntegerOverflow=on
  pdot qdot rdot : Outport  OutDataTypeStr=double  VectorParamsAs1DForOutWhenUnconnected=off
  p q  r : Outport  Port=2
  wires:
  p q r initial condition/1 -> Integrator/2
  Integrator/1 -> p q  r/1
  Reshape/1 -> pdot qdot rdot/1, Integrator/1
  Selector/1 -> I x w/2(Inertia)
  Selector2/1 -> Product2/2
  "I, I_dot"/1 -> Selector/1, Selector2/1, Selector1/1
  p q r/1 -> 3x3 Cross Product/1, I x w1/2(p q r), I x w/1(p q r)
  Product2/1 -> Reshape/1
  Sum2/1 -> Reshape1/1
  Moments/1 -> Sum2/1
  I x w1/1(Id * w) -> Sum2/2
  Selector1/1 -> I x w1/1(I_dot)
  I x w/1(I * w) -> 3x3 Cross Product/2
  Reshape1/1 -> Product2/1
  3x3 Cross Product/1 -> Sum2/3

== system lunar_lander_sim_PWPF_transferMatrix_2023a/Subsystem2/Calculate Attitude  ==
  p q r : Inport
  "phi theta psi initial condition " : Inport  Port=2
  " " : Integrator  InitialConditionSource=external
  phidot thetadot psidot : shared6dofsys/DCM & Euler Angles (Euler)/phidot thetadot psidot  SystemSampleTime=-1  VariantActivationTime=update diagram  Latency=0  AutoFrameSizeCalculation=off
  "phi theta psi " : Outport
  phidot thetadot psi : Outport  Port=2
  wires:
  "phi theta psi initial condition "/1 -> " "/2
  " "/1 -> phidot thetadot psidot/2, "phi theta psi "/1
  phidot thetadot psidot/1 -> phidot thetadot psi/1, " "/1
  p q r/1 -> phidot thetadot psidot/1

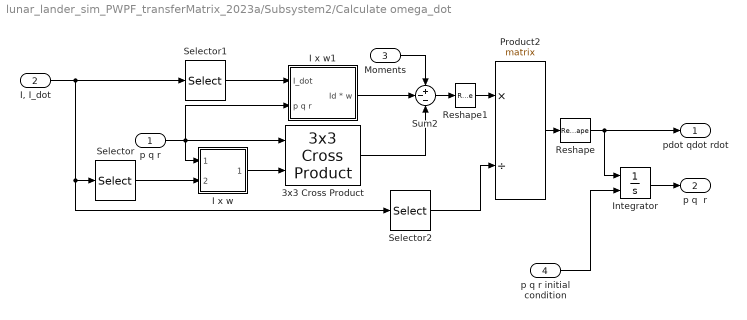
== system lunar_lander_sim_PWPF_transferMatrix_2023a/Subsystem2/Calculate omega_dot ==
  p q r : Inport  OutDataTypeStr=double
  "I, I_dot" : Inport  Port=2  OutDataTypeStr=double
  Moments : Inport  Port=3  OutDataTypeStr=double
  p q r initial condition : Inport  Port=4
  3x3 Cross Product : sharedutil/3x3 Cross Product  aMode=aMode
  I x w : Subsystem
  I x w1 : Subsystem
  Integrator : Integrator  InitialConditionSource=external
  Product2 : Product  Inputs=*/  Multiplication=Matrix(*)  SaturateOnIntegerOverflow=on  OutDataTypeStr=Inherit: Same as first input
  Reshape : Reshape
  Reshape1 : Reshape  OutputDimensionality=Row vector (2-D)
  Selector : Selector  NumberOfDimensions=2  InputPortWidth=2  IndexOptions=Index vector (dialog),Select all  Indices=1:3,-1  OutputSizes=1
  Selector1 : Selector  NumberOfDimensions=2  InputPortWidth=2  IndexOptions=Index vector (dialog),Select all  Indices=4:6,-1  OutputSizes=1
  Selector2 : Selector  NumberOfDimensions=2  InputPortWidth=2  IndexOptions=Index vector (dialog),Select all  Indices=1:3,-1  OutputSizes=1
  Sum2 : Sum  Inputs=+--  SaturateOnIntegerOverflow=on
  pdot qdot rdot : Outport  OutDataTypeStr=double  VectorParamsAs1DForOutWhenUnconnected=off
  p q  r : Outport  Port=2
  wires:
  p q r initial condition/1 -> Integrator/2
  Integrator/1 -> p q  r/1
  Reshape/1 -> pdot qdot rdot/1, Integrator/1
  Selector/1 -> I x w/2(Inertia)
  Selector2/1 -> Product2/2
  "I, I_dot"/1 -> Selector/1, Selector2/1, Selector1/1
  p q r/1 -> 3x3 Cross Product/1, I x w1/2(p q r), I x w/1(p q r)
  Product2/1 -> Reshape/1
  Sum2/1 -> Reshape1/1
  Moments/1 -> Sum2/1
  I x w1/1(Id * w) -> Sum2/2
  Selector1/1 -> I x w1/1(I_dot)
  I x w/1(I * w) -> 3x3 Cross Product/2
  Reshape1/1 -> Product2/1
  3x3 Cross Product/1 -> Sum2/3

== system lunar_lander_sim_PWPF_transferMatrix_2023a/Subsystem1/Calculate omega_dot/I x w ==
  p q r : Inport
  Inertia : Inport  Port=2
  Product : Product  Multiplication=Matrix(*)  InputSameDT=on  SaturateOnIntegerOverflow=on  OutDataTypeStr=Inherit: Same as first input
  Reshape1 : Reshape  OutputDimensionality=Column vector (2-D)
  Reshape2 : Reshape
  I * w : Outport  VectorParamsAs1DForOutWhenUnconnected=off
  wires:
  Product/1 -> Reshape2/1
  Inertia/1 -> Product/1
  p q r/1 -> Reshape1/1
  Reshape1/1 -> Product/2
  Reshape2/1 -> I * w/1

== system lunar_lander_sim_PWPF_transferMatrix_2023a/Subsystem1/Calculate omega_dot/I x w1 ==
  I_dot : Inport
  p q r : Inport  Port=2
  Product : Product  Multiplication=Matrix(*)  InputSameDT=on  SaturateOnIntegerOverflow=on  OutDataTypeStr=Inherit: Same as first input
  Reshape1 : Reshape  OutputDimensionality=Column vector (2-D)
  Reshape2 : Reshape
  Id * w : Outport  VectorParamsAs1DForOutWhenUnconnected=off
  wires:
  p q r/1 -> Reshape1/1
  I_dot/1 -> Product/1
  Product/1 -> Reshape2/1
  Reshape1/1 -> Product/2
  Reshape2/1 -> Id * w/1

== system lunar_lander_sim_PWPF_transferMatrix_2023a/Subsystem2/Calculate omega_dot/I x w ==
  p q r : Inport
  Inertia : Inport  Port=2
  Product : Product  Multiplication=Matrix(*)  InputSameDT=on  SaturateOnIntegerOverflow=on  OutDataTypeStr=Inherit: Same as first input
  Reshape1 : Reshape  OutputDimensionality=Column vector (2-D)
  Reshape2 : Reshape
  I * w : Outport  VectorParamsAs1DForOutWhenUnconnected=off
  wires:
  Product/1 -> Reshape2/1
  Inertia/1 -> Product/1
  p q r/1 -> Reshape1/1
  Reshape1/1 -> Product/2
  Reshape2/1 -> I * w/1

== system lunar_lander_sim_PWPF_transferMatrix_2023a/Subsystem2/Calculate omega_dot/I x w1 ==
  I_dot : Inport
  p q r : Inport  Port=2
  Product : Product  Multiplication=Matrix(*)  InputSameDT=on  SaturateOnIntegerOverflow=on  OutDataTypeStr=Inherit: Same as first input
  Reshape1 : Reshape  OutputDimensionality=Column vector (2-D)
  Reshape2 : Reshape
  Id * w : Outport  VectorParamsAs1DForOutWhenUnconnected=off
  wires:
  p q r/1 -> Reshape1/1
  I_dot/1 -> Product/1
  Product/1 -> Reshape2/1
  Reshape1/1 -> Product/2
  Reshape2/1 -> Id * w/1
